simulink model "sim_instalacja_podlogowa_modele"  (R2021b)
settings: Solver=VariableStepAuto  StartTime=0.0  StopTime=10.0  MaxStep=1  RelTol=1e-3
undefined symbols (not defined in the file): czas_skoku_10pro, dspr, k, T0_dwupunkt, T0_klasyczna, T_dwupunkt, T_klasyczna
settings Model: Creator=adams  LastModifiedBy=adams

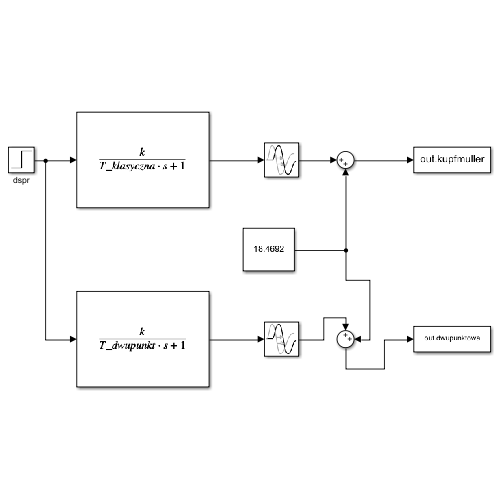
[thumbnail: Simulink's stored preview of the top-level diagram]
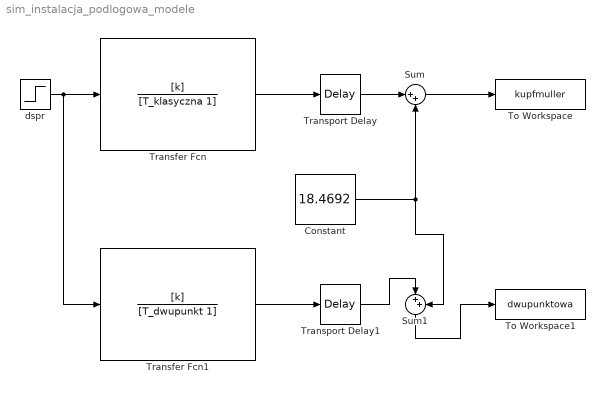
== system sim_instalacja_podlogowa_modele ==
  Constant : Constant  Value=18.4692
  Sum : Sum  Inputs=|++
  Sum1 : Sum  Inputs=|++
  To Workspace : ToWorkspace  VariableName=kupfmuller  SampleTime=-1
  To Workspace1 : ToWorkspace  VariableName=dwupunktowa  SampleTime=-1
  Transfer Fcn : TransferFcn  Numerator=[k]  Denominator=[T_klasyczna 1]
  Transfer Fcn1 : TransferFcn  Numerator=[k]  Denominator=[T_dwupunkt 1]
  Transport Delay : TransportDelay  DelayTime=T0_klasyczna  BufferSize=32768
  Transport Delay1 : TransportDelay  DelayTime=T0_dwupunkt  BufferSize=32768
  dspr : Step  Time=czas_skoku_10pro  After=dspr  SampleTime=0
  wires:
  Transport Delay/1 -> Sum/1
  Transfer Fcn1/1 -> Transport Delay1/1
  Transport Delay1/1 -> Sum1/1
  Constant/1 -> Sum/2, Sum1/2
  Transfer Fcn/1 -> Transport Delay/1
  Sum1/1 -> To Workspace1/1
  Sum/1 -> To Workspace/1
  dspr/1 -> Transfer Fcn1/1, Transfer Fcn/1
